simulink model "uz_3ph_ParameterID"  (R2022b)
settings: Solver=FixedStepDiscrete  StartTime=0.0  StopTime=160  FixedStep=0.000005  RelTol=1e-3  EnableMultiTasking=on
model workspace (MATLAB code in the model file):
  | cmdLim = Simulink.Parameter;
  | cmdLim.Value = 15;
  | cmdLim.Description = 'Limit for controlling the maximum surface command angle.';
  | cmdLim.Min = 0;
  | cmdLim.Max = 90;
  | cmdLim.DocUnits = 'deg';
  | 
  | dispGain = Simulink.Parameter;
  | dispGain.Value = 0.75;
  | dispGain.Description = 'Gain applied to the displacement error.';
  | dispGain.Min = 0;
  | dispGain.Max = [];
  | dispGain.DocUnits = 'deg/sec/deg';
  | 
  | dispLim = Simulink.Parameter;
  | dispLim.Value = 30;
  | dispLim.Description = 'Limit for controlling the maximum commanded angle.';
  | dispLim.Min = 0;
  | dispLim.Max = 180;
  | dispLim.DocUnits = 'deg';
  | 
  | intGain = Simulink.Parameter;
  | intGain.Value = 0.5;
  | intGain.Description = 'Gain applied to the integral error.';
  | intGain.Min = 0;
  | intGain.Max = [];
  | intGain.DocUnits = 'deg/sec/deg/sec';
  | 
  | intLim = Simulink.Parameter;
  | intLim.Value = 5;
  | intLim.Description = 'Limit for controlling the maximum commanded angle.';
  | intLim.Min = 0;
  | intLim.Max = 90;
  | intLim.DocUnits = 'deg';
  | 
  | rateGain = Simulink.Parameter;
  | rateGain.Value = 2;
  | rateGain.Description = 'Gain applied to the rate error.';
  | rateGain.Min = 0;
  | rateGain.Max = [];
  | rateGain.DocUnits = 'deg/deg/sec';
  | 
  | rateLim = Simulink.Parameter;
  | rateLim.Value = 6;
  | rateLim.Description = 'Limit for controlling the maximum commanded angle.';
  | rateLim.Min = 0;
  | rateLim.Max = 180;
  | rateLim.DocUnits = 'deg/sec';
  | 
  | hdgGain = Simulink.Parameter;
  | hdgGain.Value = 0.015;
values from neighbouring files (symbols this model uses):
  d_d_TMS = 0.005    [Parameter_Init_Buehler_201.m]
  d_f_hardware = 200000    [Parameter_Init_Buehler_201.m]
  d_f_states = 20000    [Parameter_Init_Buehler_201.m]
  d_i_max = 15    [Parameter_Init_Buehler_201.m]
  d_i_min = -d_i_max    (= -15)    [Parameter_Init_Buehler_201.m]
  d_I_n = 8    [Parameter_Init_Buehler_201.m]
  d_J_Coupling_M_E = 2e-6    (= 2e-06)    [Parameter_Init_Buehler_201.m]
  d_J_Coupling_M_Ms = 2e-20    [Parameter_Init_Buehler_201.m]
  d_J_Ms_L = d_J_Ms_M    (= 1.26363648e-05)    [Parameter_Init_Buehler_201.m]
  d_J_Ms_M = 0.5*0.5*((0.5*d_d_Ms)^4)*3.14*d_l_Ms*d_rho_Ms    (= 1.26363648e-05)    [Parameter_Init_Buehler_201.m]
  d_L_d = 0.00031    [Parameter_Init_Buehler_201.m]
  d_L_q = 0.00033    [Parameter_Init_Buehler_201.m]
  d_p = 4    [Parameter_Init_Buehler_201.m]
  d_psi_pm = 0.0075    [Parameter_Init_Buehler_201.m]
  d_R_ph = d_R_ph_ph/2    (= 0.089)    [Parameter_Init_Buehler_201.m]
  d_y_max = 10    [Parameter_Init_Buehler_201.m]
  d_y_min = -d_y_max    (= -10)    [Parameter_Init_Buehler_201.m]
undefined symbols (not defined in the file or in its folder): i_dq, i_dq_ref, n_ref, V_abc, v_dq
libraries: fl_lib x47, nesl_utility x30, ee_lib x18, simulink x8, spsabctodq0Lib x2, spsdq0toabcLib x1, spsTriangleGeneratorLib x1
(part 1 of 4)
settings Model: RequirementInfo={} %GIDa_fe9045fd_0412_4b6e_8206_617cc20e6fde  FPTRunName=Active  Creator=ts  LastModifiedBy=valen
settings SolverCC: AlgebraicLoopSolver=TrustRegion  PositivePriorityOrder=on  AutoInsertRateTranBlk=on
settings DataIOCC: SaveOutput=off  SignalLogging=off  DSMLogging=off  SaveTime=off
settings OptimizationCC: DefaultParameterBehavior=Inlined  UseDivisionForNetSlopeComputation=on  GainParamInheritBuiltInType=on  UseFloatMulNetSlope=on  DefaultUnderspecifiedDataType=single  UseSpecifiedMinMax=on  InlineInvariantSignals=on  PassReuseOutputArgsAs=Individual arguments  ZeroExternalMemoryAtStartup=off  ZeroInternalMemoryAtStartup=off  NoFixptDivByZeroProtection=on  EfficientFloat2IntCast=on  LifeSpan=1  MaxStackSize=64  OptimizeBlockOrder=speed  DifferentSizesBufferReuse=on  EfficientTunableParamExpr=on
settings DebuggingCC: UnconnectedInputMsg=warning  UnconnectedOutputMsg=warning  UnconnectedLineMsg=warning  BusObjectLabelMismatch=error  AllowSymbolicDim=off  SFUnexpectedBacktrackingDiag=warning  SFNoUnconditionalDefaultTransitionDiag=warning  SFExecutionAtInitializationDiag=none  SFMachineParentedDataDiag=warning  ArithmeticOperatorsInVariantConditions=warning
settings HardwareCC: ProdBitPerPointer=32  ProdBitPerSizeT=32  ProdBitPerPtrDiffT=32  ProdLargestAtomicInteger=Long  ProdLargestAtomicFloat=Double  ProdWordSize=32  ProdLongLongMode=on  ProdHWDeviceType=ARM Compatible->ARM Cortex-R  HardwareBoardFeatureSet=SoCBlockset
settings ModelReferenceCC: EnableRefExpFcnMdlSchedulingChecks=on
settings SFSimCC: SimGenImportedTypeDefs=on  MATLABDynamicMemAlloc=off
settings RTWCC: Description=Embedded Coder  SystemTargetFile=ert.tlc  GenCodeOnly=on  TemplateMakefile=ert_default_tmf  GenerateReport=on  BuildConfiguration=Faster Runs  IncludeHyperlinkInReport=on  LaunchReport=on  GenerateTraceInfo=on  GenerateTraceReport=on  GenerateTraceReportSl=on  GenerateTraceReportSf=on  GenerateTraceReportEml=on  GenerateCodeMetricsReport=on  CheckMdlBeforeBuild=Warning  DLArmComputeVersion=19.05
settings CodeAppCC: ForceParamTrailComments=on  IgnoreCustomStorageClasses=off  OperatorAnnotations=on  SimulinkDataObjDesc=on  SFDataObjDesc=on  MATLABFcnDesc=on  CustomSymbolStrGlobalVar=rt$M$R$N  CustomSymbolStrType=$N$M$R_t  CustomSymbolStrFcn=$N$M$F  CustomSymbolStrMacro=$N$M  InsertBlockDesc=on  StateflowObjectComments=on  MATLABSourceComments=on  EnableCustomComments=on  ReqsInCode=on
settings ERTTargetCC: TargetLangStandard=C99 (ISO)  CodeReplacementLibrary=GNU C99 extensions  MultiwordLength=2048  IncludeMdlTerminateFcn=off  CombineSignalStateStructs=on  SuppressErrorStatus=on  IncludeFileDelimiter=UseQuote  CodeInterfacePackaging=Reusable function  SupportNonFinite=off  RemoveResetFunc=off  InlinedParameterPlacement=NonHierarchical  MultiInstanceErrorCode=Warning  RootIOFormat=Part of model data structure  ERTCustomFileTemplate=example_file_process.tlc  GlobalDataDefinition=InSourceFile  GlobalDataReference=InSourceFile  ERTFilePackagingFormat=CompactWithDataFile  SuppressUnreachableDefaultCases=off
settings ConfigComp: CovScope=ReferencedModels  CovSaveName=covdata_rollAP  CovMetricSettings=dcmtrwe  CovHTMLOptions=-sRT=1 -aTS=1 -bRG=1 -bTC=1 -hTR=1 -nFC=0 -scm=1 -bcm=1 -xEv=0  CovSaveCumulativeToWorkspaceVar=on  CovSaveSingleToWorkspaceVar=on  CovCumulativeVarName=covCumulativeData_rollAP  CovReportOnPause=off  CovExternalEMLEnable=off  CovSFcnEnable=off

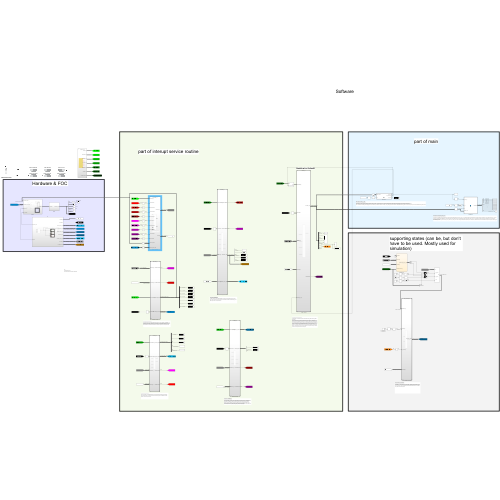
[thumbnail: Simulink's stored preview of the top-level diagram]
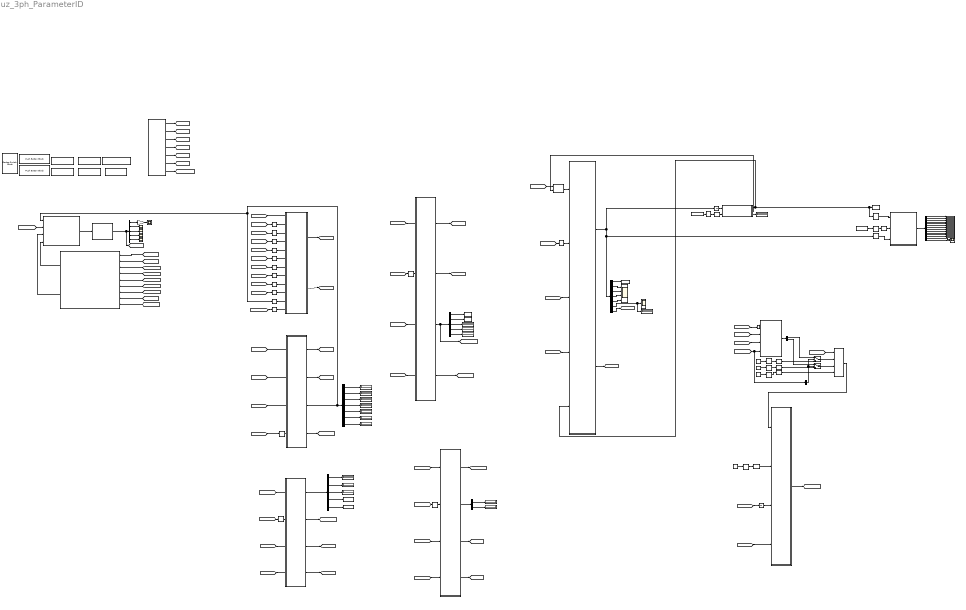
== system uz_3ph_ParameterID ==
  note: todo:
      | -control state reference
      | -two mass generieren mit externen definitionen
  note: Description of Interpoaltion_Mesh_Grid:
      |
      | This function is calculating the regular flux maps out of the irregular scatter data array stored in psi_array_in. The outputs rangeX are containg the flux maps axis information, whereby the range is related to 3 times "i_rat" input.
      | Furthermore, the temperature dependency of the permanent flux is calculated if there are enough measuring values stored in the "delta_psi" array. The temperature constant as well as the estimated error of permanent flux,
      | at reference temperature, are given out on "psi_temp_const" and "psi_temp_error" outputs. Using this temperature dependency, the flux maps are updated with the permanent flux offset caused by the temperature which is given
      | in on "Wtemp_in" input.
  note: Stateflow for OnlineID
  note: part of main
  note: part of interupt service routine
  note: Software
  note: Hardware & FOC
  note: Description of clean_psi_array:
      |
      | This function is cleaning the array storing the measurement values, which always consits of a d-q-current combination a winding temperature and a speed value such as a d-q-flux combination
      | The function is searching for measuring pairs which are closer than "eta_c" to their neighbours. In this case it is averaging this similar pairs to avoid measuring values containing the same information.
      | This is essential for calculating a wide ranging flux map out of this array. Furthermore, there is an output "n_flux_points" giving back the amount of independent measuring pairs. This is the number (x/100) i show in the JavaGUI on the rigth top corner.
  note: Description of ElectricalID:
      |
      | This state includes an automated identification process for typical parameters of a PMSM. This includes the identification of the polepairs, theta_offset of a incremental encoder, Rs, Ld, Lq, Psi_PM and J. The control parameters of a FOC will be calculated with the identified parameters and are therefore tuned for the used machine. This state requires some sort of speed control.
  note: Description OnlineID Stateflow:
      |
      | This Stateflow is used to detect special transient states and to gather measuring data in these states.
      | This is done to identify the parameters of the linear pmsm model. This includes Rs, Ld, Lq and Psi_PM. The flux maps can be identified aswell. With each new operating point the relevant signals are measured and the flux in the specific operating point is calculated. Up to 100 unique values will be stored in an array, which will later be cleaned up with external functions. In contrast to the FluxMapID state, this state does not actively control the machine via reference currents(except the addition of a injection signal with low amplitude/frequency on top of the reference d-axis current), but therefore measures and calculates the flux in the operating points. This state can therefore run in parallel with your controller, since it does not require full control of the system.
  note: Description of FrictionID:
      |
      | This state includes an automated identification process for different friction/torque parameters. The breakaway torque, coloumb torque and viscous friction torque will be identified. This state requires some sort of speed control.
  note: Description of FluxMapID:
      |
      | This state includes an process for FluxMap identification. The desired range of the identified flux maps can be set in the d- and q-axis, with an input for the stepsize aswell. From these input parameters, this state will create a rectangular grid. Each point of this grid will be set and reference currents outputed to an external current controller. This state needs some sort of current controller to work properly. It does NOT measure the needed signals to calculate the flux maps in each point. It only controls the triggering of the operating points.
  note: Description of TwoMassID:
      |
      | This state includes an automated identification process for typical parameters of a two mass system. This includes the inertia of the motor and load side, the stiffness and the damping. This state requires some sort of speed control.
  note: Description FOC_ControlState:
      |
      | This Stateflow is entered, after every other ID-state is finished (except OnlineID). It's just a simple state for current & speed control, depending on what the user chose in the config. This is only used to control the FOC with inputs after the ID-states are done. This state is solely used for simulation purposes.
  note: supporting states (can be, but don't have to be used. Mostly used for simulation)
  0 = current control 1 = speed control : Constant
  AutoRefCurrents : Stateflow chart  TreatAsAtomicUnit=on
      settings: PortSchema="{\"entries\":[{\"content\":{\"sides\":[{\"content\":{\"connectorIds\":[\"In1\",\"In2\",\"In4\",\"In3\"]},\"type\":\"ConnectorPlacement.EquallySpacedRectSide\",\"uuid\":\"72ec0a24-315d-4dd0-9768-288ce3b452e0\"},{\"content\":{\"connectorIds\":[\"Out1\"],\"side\":\"RIGHT\"},\"type\":\"ConnectorPlacement.EquallySpacedRectSide\",\"uuid\":\"ab2b6233-d9cb-4afd-91e6-1fd664e04fd4\"},{\"content\":{\"connectorIds\":[],\"side\":\"TOP\"},\"type\":\"ConnectorPlacement.EquallySpacedRectSide\",\"uuid\":\"64b2df27-0928-499d-b44c-d4351b3511f9\"}]},\"type\":\"ConnectorPlacement.EquallySpacedConnector\",\"uuid\":\"4bb55e1f-14f7-4ef2-bb52-ee940a9b3e5d\"}],\"packageUris\":[\"http://schema.mathworks.com/mf0/Connector/R2020b\"],\"version\":\"1.0\"}"
  Bus Assignment : BusAssignment  AssignedSignals=i_dq_ref.d,i_dq_ref.q,n_ref
  Bus Assignment1 : BusAssignment  AssignedSignals=array_cleaned
  Bus Selector : BusSelector  OutputSignals=BrkTorque,CoulTorque,ViscoTorque,measArrayTorque,measArraySpeed
  Bus Selector1 : BusSelector  OutputSignals=omega_m,i_dq,v_dq,I_abc,V_abc
  Bus Selector2 : BusSelector  OutputSignals=thetaOffset,PMSM_parameters.R_ph_Ohm,PMSM_parameters.Ld_Henry,PMSM_parameters.Lq_Henry,PMSM_parameters.Psi_PM_Vs,PMSM_parameters.J_kg_m_squared,PMSM_parameters.polePairs
  Bus Selector3 : BusSelector  OutputSignals=range_psid_X,range_psiq_X,range_id_X,range_iq_X,range_psid_Y,range_psiq_Y,range_id_Y,range_iq_Y,psiq_grid,psid_grid,id_grid,iq_grid,psi_temp_const,psi_temp_error
  Bus Selector4 : BusSelector  OutputSignals=i_dq_ref.d,i_dq_ref.q
  Bus Selector5 : BusSelector  OutputSignals=R_s,WindingTemp
  Bus Selector6 : BusSelector  OutputSignals=c_est_out,d_est_out,LoadInertia,TrainInertia,rotorInertia
  Bus Selector7 : BusSelector  OutputSignals=enableCRS
  Bus Selector8 : BusSelector  OutputSignals=psi_array,Rph_out,Ld_out,Lq_out,psi_pm_out,activeState,id_out
  CleanPsiArray : MATLAB Function
  Const27 : Constant  Value=0.01*d_I_n
  Const53 : Constant  Value=d_I_n
  Const7 : Constant  Value=0.6
  Const8 : Constant  Value=0
  Const9 : Constant  Value=1000
  Data Type Conversion107 : DataTypeConversion  OutDataTypeStr=boolean  SaturateOnIntegerOverflow=off  RndMeth=Floor
  Data Type Conversion{12..13,15,60,86} (5 alike) : DataTypeConversion  OutDataTypeStr=single  SaturateOnIntegerOverflow=off  RndMeth=Floor
  Delay{,1..9,14} (11 alike) : Delay  DelayLength=1  InitialCondition=0
  Display{1..3,5..11} (10 alike) : Display
  ElectricalID_subsystem : ModelReference  ModelNameDialog=ElectricalID_ref.slx  SimulationMode=Normal  ModelReferenceVersion=5.61
      settings: PortSchema="{\"entries\":[{\"content\":{\"sides\":[{\"content\":{\"connectorIds\":[\"In3\",\"In4\",\"In1\",\"In2\"]},\"type\":\"ConnectorPlacement.EquallySpacedRectSide\",\"uuid\":\"f0ac0bcf-14d9-46a0-98b5-cf926ef17a03\"},{\"content\":{\"connectorIds\":[\"Out1\",\"Out2\",\"Out4\",\"Out3\"],\"side\":\"RIGHT\"},\"type\":\"ConnectorPlacement.EquallySpacedRectSide\",\"uuid\":\"3432f655-d87e-4f4a-bc13-594c8277a670\"},{\"content\":{\"connectorIds\":[],\"side\":\"TOP\"},\"type\":\"ConnectorPlacement.EquallySpacedRectSide\",\"uuid\":\"598e67a2-ee08-4059-aaa7-0b5cb688c228\"}]},\"type\":\"ConnectorPlacement.EquallySpacedConnector\",\"uuid\":\"e19c3dd0-4872-4ea8-9ebd-fc7e1d9ddc42\"}],\"packageUris\":[\"http://schema.mathworks.com/mf0/Connector/R2020b\"],\"version\":\"1.0\"}"
  FOC : Subsystem
  FOC_ControlState_subsystem : ModelReference  ModelNameDialog=FOC_ControlState_ref.slx  SimulationMode=Normal  ModelReferenceVersion=5.47
      settings: PortSchema="{\"entries\":[{\"content\":{\"sides\":[{\"content\":{\"connectorIds\":[\"In2\",\"In4\",\"In1\",\"In3\"]},\"type\":\"ConnectorPlacement.EquallySpacedRectSide\",\"uuid\":\"51616e24-a97c-4867-a832-fbf8995ba5af\"},{\"content\":{\"connectorIds\":[\"Out1\"],\"side\":\"RIGHT\"},\"type\":\"ConnectorPlacement.EquallySpacedRectSide\",\"uuid\":\"f89ef2d6-1fe7-4143-9573-492fc01180c7\"},{\"content\":{\"connectorIds\":[],\"side\":\"TOP\"},\"type\":\"ConnectorPlacement.EquallySpacedRectSide\",\"uuid\":\"2a1663ee-9e4b-4188-8f87-b811d0bf4173\"}]},\"type\":\"ConnectorPlacement.EquallySpacedConnector\",\"uuid\":\"7415555a-a8a9-4dd7-91ae-86382220971a\"}],\"packageUris\":[\"http://schema.mathworks.com/mf0/Connector/R2020b\"],\"version\":\"1.0\"}"
  FluxMapID_subsystem : ModelReference  ModelNameDialog=FluxMapID_ref.slx  SimulationMode=Normal  ModelReferenceVersion=5.45
      settings: PortSchema="{\"entries\":[{\"content\":{\"sides\":[{\"content\":{\"connectorIds\":[\"In1\",\"In2\",\"In3\",\"In4\"]},\"type\":\"ConnectorPlacement.EquallySpacedRectSide\",\"uuid\":\"981d5bbf-03cd-4404-8840-685ce2b7a497\"},{\"content\":{\"connectorIds\":[\"Out3\",\"Out4\",\"Out1\",\"Out2\"],\"side\":\"RIGHT\"},\"type\":\"ConnectorPlacement.EquallySpacedRectSide\",\"uuid\":\"92ae37cc-cac4-4d7b-af20-0fade983881b\"},{\"content\":{\"connectorIds\":[],\"side\":\"TOP\"},\"type\":\"ConnectorPlacement.EquallySpacedRectSide\",\"uuid\":\"d233b8d0-893b-4073-8e4e-3204ab89fedb\"}]},\"type\":\"ConnectorPlacement.EquallySpacedConnector\",\"uuid\":\"28ed47dd-3acf-49aa-8a06-7eb7a90c4cf1\"}],\"packageUris\":[\"http://schema.mathworks.com/mf0/Connector/R2020b\"],\"version\":\"1.0\"}"
  FrictionID_subsystem : ModelReference  ModelNameDialog=FrictionID_ref.slx  SimulationMode=Normal  ModelReferenceVersion=5.45
      settings: PortSchema="{\"entries\":[{\"content\":{\"sides\":[{\"content\":{\"connectorIds\":[\"In1\",\"In2\",\"In3\",\"In4\"]},\"type\":\"ConnectorPlacement.EquallySpacedRectSide\",\"uuid\":\"9228c284-4dde-45fc-9186-6f631f78e5bf\"},{\"content\":{\"connectorIds\":[\"Out4\",\"Out3\",\"Out2\",\"Out1\"],\"side\":\"RIGHT\"},\"type\":\"ConnectorPlacement.EquallySpacedRectSide\",\"uuid\":\"71961043-480b-43aa-8cdd-23d9057d5ad4\"},{\"content\":{\"connectorIds\":[],\"side\":\"TOP\"},\"type\":\"ConnectorPlacement.EquallySpacedRectSide\",\"uuid\":\"f6f3bc9d-566f-4498-bf43-24e8b901b7a7\"}]},\"type\":\"ConnectorPlacement.EquallySpacedConnector\",\"uuid\":\"83d2d7c4-30d1-4ed4-b102-cbae6a0e9817\"}],\"packageUris\":[\"http://schema.mathworks.com/mf0/Connector/R2020b\"],\"version\":\"1.0\"}"
  Gain : Gain  Gain=60/(2*pi)
  Hardware : Subsystem
  I_abc : Scope
  InterpMeshGrid : MATLAB Function  TreatAsAtomicUnit=on
  OnlineActiveState : Scope
  OnlineID_subsystem : ModelReference  ModelNameDialog=OnlineID_ref.slx  SimulationMode=Normal  ModelReferenceVersion=5.46
      settings: PortSchema="{\"entries\":[{\"content\":{\"sides\":[{\"content\":{\"connectorIds\":[\"In2\",\"In3\",\"In4\",\"In5\",\"In1\"]},\"type\":\"ConnectorPlacement.EquallySpacedRectSide\",\"uuid\":\"7820c6f2-c977-4194-b662-7782d124a170\"},{\"content\":{\"connectorIds\":[\"Out1\",\"Out2\"],\"side\":\"RIGHT\"},\"type\":\"ConnectorPlacement.EquallySpacedRectSide\",\"uuid\":\"8a942b25-9a71-4f6d-9e71-d8e23af023a4\"},{\"content\":{\"connectorIds\":[],\"side\":\"TOP\"},\"type\":\"ConnectorPlacement.EquallySpacedRectSide\",\"uuid\":\"547238ca-03bf-4702-a4be-178f97463404\"}]},\"type\":\"ConnectorPlacement.EquallySpacedConnector\",\"uuid\":\"69f1930a-cf81-42da-9647-066ad6599903\"}],\"packageUris\":[\"http://schema.mathworks.com/mf0/Connector/R2020b\"],\"version\":\"1.0\"}"
  Push Button2 : PushButtonBlock  ButtonText=RESET
  Push Button3 : PushButtonBlock  ButtonText=ACCEPT  OffValue=1.000000
  RT : RateTransition  OutPortSampleTime=0.0001
  Rate Transition : RateTransition  OutPortSampleTime=0.1
  Rate Transition{1..6,13..14,78,147} (10 alike) : RateTransition  OutPortSampleTime=1/d_f_states
  Rate Transition85 : RateTransition  OutPortSampleTime=0.1
  Rate Transition90 : RateTransition  OutPortSampleTime=0.1
  Rs,Ld,Lq,Psi_pm : Scope  NumInputPorts=4
  Scope2 : Scope  NumInputPorts=2
  Select Control : SliderSwitchBlock  LabelPosition=Hide
      settings: Values={{'Current', 'Speed'}, [0 1]}
  Subsystem Reference : Subsystem  ReferencedSubsystem=model_bus_init
  Subsystem Reference1 : Subsystem  ReferencedSubsystem=ControlState_ref
  Switch2 : Switch  Criteria=u2 > Threshold  SaturateOnIntegerOverflow=off  InputSameDT=off
  Switch3 : Switch  Criteria=u2 > Threshold  SaturateOnIntegerOverflow=off  InputSameDT=off
  To Workspace1 : ToWorkspace  VariableName=measArrayTorque  SampleTime=-1
      settings: MaxDataPoints=1
  To Workspace15 : ToWorkspace  VariableName=psi_array_cleaned  SampleTime=-1
      settings: MaxDataPoints=1
  To Workspace16 : ToWorkspace  VariableName=rangepdX  SampleTime=-1
      settings: MaxDataPoints=1
  To Workspace17 : ToWorkspace  VariableName=rangepqX  SampleTime=-1
      settings: MaxDataPoints=1
  To Workspace18 : ToWorkspace  VariableName=rangeidX  SampleTime=-1
      settings: MaxDataPoints=1
  To Workspace19 : ToWorkspace  VariableName=rangeiqX  SampleTime=-1
      settings: MaxDataPoints=1
  To Workspace2 : ToWorkspace  VariableName=measArraySpeed  SampleTime=-1
      settings: MaxDataPoints=1
  To Workspace20 : ToWorkspace  VariableName=rangepdY  SampleTime=-1
      settings: MaxDataPoints=1
  To Workspace21 : ToWorkspace  VariableName=rangepqY  SampleTime=-1
      settings: MaxDataPoints=1
  To Workspace22 : ToWorkspace  VariableName=rangeidY  SampleTime=-1
      settings: MaxDataPoints=1
  To Workspace23 : ToWorkspace  VariableName=rangeiqY  SampleTime=-1
      settings: MaxDataPoints=1
  To Workspace24 : ToWorkspace  VariableName=psiq_grid  SampleTime=-1
      settings: MaxDataPoints=1
  To Workspace25 : ToWorkspace  VariableName=psid_grid  SampleTime=-1
      settings: MaxDataPoints=1
  To Workspace26 : ToWorkspace  VariableName=id_grid  SampleTime=-1
      settings: MaxDataPoints=1
  To Workspace27 : ToWorkspace  VariableName=iq_grid  SampleTime=-1
      settings: MaxDataPoints=1
  To Workspace3 : ToWorkspace  VariableName=psi_array  SampleTime=-1
      settings: MaxDataPoints=1
  To Workspace31 : ToWorkspace  VariableName=c_est_out  SampleTime=-1
      settings: MaxDataPoints=1
  To Workspace32 : ToWorkspace  VariableName=d_est_out  SampleTime=-1
      settings: MaxDataPoints=1
  TwoMassID_subsystem : ModelReference  ModelNameDialog=TwoMassID_ref.slx  SimulationMode=Normal  ModelReferenceVersion=5.45
      settings: PortSchema="{\"entries\":[{\"content\":{\"sides\":[{\"content\":{\"connectorIds\":[\"In1\",\"In2\",\"In3\",\"In4\"]},\"type\":\"ConnectorPlacement.EquallySpacedRectSide\",\"uuid\":\"b3f846b4-67b8-414d-80f8-2cdf230e8050\"},{\"content\":{\"connectorIds\":[\"Out1\",\"Out2\",\"Out4\",\"Out3\"],\"side\":\"RIGHT\"},\"type\":\"ConnectorPlacement.EquallySpacedRectSide\",\"uuid\":\"f153ecc1-7a63-46b5-bb71-72b88e4117b7\"},{\"content\":{\"connectorIds\":[],\"side\":\"TOP\"},\"type\":\"ConnectorPlacement.EquallySpacedRectSide\",\"uuid\":\"7aaf7a4c-17fe-4dd1-8ce1-675b09504e17\"}]},\"type\":\"ConnectorPlacement.EquallySpacedConnector\",\"uuid\":\"e21480e7-4483-4a1e-b62d-5327482c3f88\"}],\"packageUris\":[\"http://schema.mathworks.com/mf0/Connector/R2020b\"],\"version\":\"1.0\"}"
  Unit Delay : UnitDelay  SampleTime=-1  HasFrameUpgradeWarning=on
  Unit Delay3 : UnitDelay  SampleTime=-1  HasFrameUpgradeWarning=on
  V_abc : Scope
  d-axis inductance Ld [H] : Display
  dqTrans : Subsystem
  enable ElectricalID : SliderSwitchBlock  LabelPosition=Hide
      settings: Values={{'Off', 'On'}, [0 1]}
  enable FluxMapID : SliderSwitchBlock  LabelPosition=Hide
      settings: Values={{'Off', 'On'}, [0 1]}
  enable FrictionID : SliderSwitchBlock  LabelPosition=Hide
      settings: Values={{'Off', 'On'}, [0 1]}
  enable OnlineID : SliderSwitchBlock  LabelPosition=Hide
      settings: Values={{'Off', 'On'}, [0 1]}
  enable TwoMassID : SliderSwitchBlock  LabelPosition=Hide
      settings: Values={{'Off', 'On'}, [0 1]}
  enableParameterID : RockerSwitchBlock  LabelPosition=Hide
      settings: Values={{'Off', 'On'}, [0 1]}
  i_d i_q : Scope
  p : Display
  phase resistance [Ohm] : Display
  psiPM [Vs] : Display
  q-axis inductance Lq [H] : Display
  rotor speed [rpm] : Scope
  rotorInertia  [kg*m²] : Display
  thetaOffset [rad] : Display
  v_d v_q : Scope
  wires:
  FrictionID_subsystem/1 -> [finishedFrictionID]
  Bus Selector/3 -> Display10/1  "<ViscoTorque>"
  FluxMapID_subsystem/1 -> [finishedFluxMapID]
  [ControlFlags] -> OnlineID_subsystem/5
  Const8/1 -> Rate Transition13/1
  Subsystem Reference/5 -> [TwoMassIDConfig]
  Bus Selector2/4 -> q-axis inductance Lq [H]/1  "<Lq_Henry>"
  [GlobalConfig] -> AutoRefCurrents/2(GlobalConfig)
  [GlobalConfig] -> FluxMapID_subsystem/3
  [finishedFrictionID] -> Delay/1
  Rate Transition5/1 -> FrictionID_subsystem/2
  TwoMassID_subsystem/4 -> [TwoMassID_output], Bus Selector6/1
  OnlineID_subsystem/1 -> Bus Selector8/1, Rate Transition90/1, Unit Delay3/1
  Bus Selector2/5 -> psiPM [Vs]/1  "<Psi_PM_Vs>"
  Gain/1 -> rotor speed [rpm]/1
  Bus Selector8/2 -> Rs,Ld,Lq,Psi_pm/1  "<Rph_out>"
  Rate Transition2/1 -> TwoMassID_subsystem/2
  ElectricalID_subsystem/3 -> [ElectricalID_FOC_output]
  Bus Selector6/5 -> Display6/1  "<rotorInertia>"
  Const9/1 -> Rate Transition1/1
  Rate Transition14/1 -> Data Type Conversion13/1
  Subsystem Reference/1 -> [GlobalConfig_in]
  ElectricalID_subsystem/4 -> Hardware/1(ElectricalID_output), Delay14/1, Bus Selector2/1
  [FrictionIDConfig] -> FrictionID_subsystem/1
  [FluxMapID_FOC_output] -> FOC/5(FluxMapID_FOC_input)
  [enteredElectricalID] -> Delay5/1
  ElectricalID_subsystem/1 -> [enteredElectricalID]
  Rate Transition85/1 -> Data Type Conversion86/1
  [enteredFrictionID] -> Delay1/1
  [FOCControl_output] -> FOC/6(FOCControl_input)
  FluxMapID_subsystem/4 -> Bus Selector5/1
  Data Type Conversion13/1 -> Switch2/3  "i_q_ref"
  Rate Transition90/1 -> InterpMeshGrid/3(OnlineID_input)
  [finishedFluxMapID] -> Delay4/1
  ElectricalID_subsystem/2 -> [finishedElectricalID]
  [ControlFlags] -> ElectricalID_subsystem/4
  [finishedTwoMassID] -> Delay3/1
  FOC/2(PWM_out) -> Hardware/3(PWM_FOC_in)
  [ActualValues] -> RT/1
  Bus Selector1/1 -> Gain/1  "<omega_m>"
  Subsystem Reference/2 -> [ElectricalIDConfig]
  [ElectricalIDConfig] -> ElectricalID_subsystem/1
  TwoMassID_subsystem/3 -> [TwoMassID_FOC_output]
  Subsystem Reference/4 -> [FrictionIDConfig]
  Const53/1 -> Rate Transition85/1
  [GlobalConfig] -> TwoMassID_subsystem/3
  FluxMapID_subsystem/3 -> [FluxMapID_FOC_output]
  Const27/1 -> Rate Transition78/1
  [ControlFlags] -> TwoMassID_subsystem/4
  TwoMassID_subsystem/1 -> [finishedTwoMassID]
  Data Type Conversion60/1 -> CleanPsiArray/2(eta_c)
  Bus Selector2/6 -> rotorInertia  [kg*m²]/1  "<J_kg_m_squared>"
  Bus Selector/1 -> Display11/1  "<BrkTorque>"
  [TwoMassIDConfig] -> TwoMassID_subsystem/1
  Bus Selector2/7 -> p/1  "<polePairs>"
  [ElectricalID_FOC_output] -> Delay8/1
  Rate Transition13/1 -> Data Type Conversion12/1
  Unit Delay/1 -> FOC_ControlState_subsystem/1
  FrictionID_subsystem/3 -> [FrictionID_FOC_output]  "FrictionID_FOC_output"
  Rate Transition/1 -> InterpMeshGrid/1(psi_array_in)
  TwoMassID_subsystem/2 -> [enteredTwoMassID]
  Bus Selector2/2 -> phase resistance [Ohm]/1  "<R_ph_Ohm>"
  Rate Transition3/1 -> OnlineID_subsystem/3
  [GlobalConfig] -> ElectricalID_subsystem/3
  Bus Selector2/3 -> d-axis inductance Ld [H]/1  "<Ld_Henry>"
  [ActualValues] -> Rate Transition6/1
  Bus Selector6/3 -> Display3/1  "<LoadInertia>"
  [ControlFlags] -> FOC/1(ControlFlags)
  Rate Transition6/1 -> ElectricalID_subsystem/2
  [FluxMapIDConfig] -> FluxMapID_subsystem/1
  [ActualValues] -> Rate Transition2/1
  Subsystem Reference/6 -> [OnlineIDConfig]
  [ControlFlags] -> FluxMapID_subsystem/4
  [ActualValues] -> Rate Transition3/1
  CleanPsiArray/2(array_cleaned_flag) -> Bus Assignment1/2
  Bus Selector5/1 -> Display1/1  "<R_s>"
  [GlobalConfig] -> FrictionID_subsystem/3
  [ControlFlags] -> FOC_ControlState_subsystem/3
  [ElectricalID_FOC_output] -> Hardware/2(ElectricalID_FOC_output)
  Const7/1 -> Rate Transition14/1
  FrictionID_subsystem/4 -> Bus Selector/1
  FrictionID_subsystem/2 -> [enteredFrictionID]
  Bus Selector6/4 -> Display5/1  "<TrainInertia>"
  Hardware/1(ActualValues) -> dqTrans/1(ActualValues)
  Data Type Conversion86/1 -> InterpMeshGrid/2(i_rat)
  Bus Selector8/5 -> Rs,Ld,Lq,Psi_pm/4  "<psi_pm_out>"
  Bus Selector8/3 -> Rs,Ld,Lq,Psi_pm/2  "<Ld_out>"
  Unit Delay3/1 -> CleanPsiArray/1(OnlineID_output)
  [OnlineIDConfig] -> Bus Assignment1/1
  [TwoMassID_FOC_output] -> FOC/7(TwoMassID_FOC_input)
  Rate Transition78/1 -> Data Type Conversion60/1
  Rate Transition1/1 -> Data Type Conversion15/1
  Bus Selector8/6 -> Display8/1, OnlineActiveState/1  "<activeState>"
  CleanPsiArray/1(psi_array_out) -> Rate Transition/1, To Workspace15/1, OnlineID_subsystem/1  "cleaned_psi_array"
  [GlobalConfig] -> OnlineID_subsystem/4
  FOC/1(FOC_enable_out) -> Hardware/4(FOC_enabled)
  Bus Selector2/1 -> thetaOffset [rad]/1  "<thetaOffset>"
  Rate Transition4/1 -> FluxMapID_subsystem/2
  Subsystem Reference/3 -> [FluxMapIDConfig]
  [FrictionID_FOC_output] -> FOC/3(FrictionID_FOC_input)
  Bus Selector1/2 -> i_d i_q/1  "<i_dq>"
  CleanPsiArray/3(n_flux_points) -> Display7/1
  Bus Selector/2 -> Display9/1  "<CoulTorque>"
  FluxMapID_subsystem/2 -> [enteredFluxMapID]
  [ActualValues] -> Rate Transition4/1
  Bus Selector6/1 -> To Workspace31/1  "<c_est_out>"
  Bus Selector6/2 -> To Workspace32/1  "<d_est_out>"
  FOC_ControlState_subsystem/1 -> [FOCControl_output]
  [finishedElectricalID] -> Delay7/1
  [ElectricalID_FOC_output] -> FOC/4(ElectricalID_FOC_input)
  Bus Assignment/1 -> FOC_ControlState_subsystem/2
  [ControlFlags] -> FrictionID_subsystem/4
  [ActualValues] -> Rate Transition5/1
  Bus Selector8/4 -> Rs,Ld,Lq,Psi_pm/3  "<Lq_out>"
  Data Type Conversion12/1 -> Switch3/3  "i_d_ref"
  [enteredFluxMapID] -> Delay2/1
  [ActualValues] -> FOC/2(ActualValues)
  [enteredTwoMassID] -> Delay6/1
  Bus Selector5/2 -> Display2/1  "<WindingTemp>"
  Bus Selector1/3 -> v_d v_q/1  "<v_dq>"
  Bus Selector1/4 -> I_abc/1  "<I_abc>"
  Bus Selector1/5 -> V_abc/1  "<V_abc>"
  [GlobalConfig] -> Bus Assignment/1
  Switch2/1 -> Bus Assignment/3
  Switch3/1 -> Bus Assignment/2
  Data Type Conversion15/1 -> Bus Assignment/4  "n_ref"
  RT/1 -> AutoRefCurrents/1(ActualValues)
  Bus Selector8/7 -> [OnlineID_id_out]  "<id_out>"
  [OnlineID_id_out] -> Unit Delay/1
  Rate Transition147/1 -> Data Type Conversion107/1
  Data Type Conversion107/1 -> FOC_ControlState_subsystem/4  "controlType"
  0 = current control 1 = speed control/1 -> Rate Transition147/1
  Bus Assignment1/1 -> OnlineID_subsystem/2
  Bus Selector3/1 -> To Workspace16/1  "<range_psid_X>"
  Bus Selector3/2 -> To Workspace17/1  "<range_psiq_X>"
  InterpMeshGrid/1(FluxMapData) -> Bus Selector3/1
  Bus Selector3/14 -> Scope2/2  "<psi_temp_error>"
  Bus Selector3/13 -> Scope2/1  "<psi_temp_const>"
  Bus Selector3/3 -> To Workspace18/1  "<range_id_X>"
  Bus Selector3/4 -> To Workspace19/1  "<range_iq_X>"
  Bus Selector3/5 -> To Workspace20/1  "<range_psid_Y>"
  Bus Selector3/6 -> To Workspace21/1  "<range_psiq_Y>"
  Bus Selector3/7 -> To Workspace22/1  "<range_id_Y>"
  Bus Selector3/8 -> To Workspace23/1  "<range_iq_Y>"
  Bus Selector3/9 -> To Workspace24/1  "<psiq_grid>"
  Bus Selector3/10 -> To Workspace25/1  "<psid_grid>"
  Bus Selector3/11 -> To Workspace26/1  "<id_grid>"
  Bus Selector3/12 -> To Workspace27/1  "<iq_grid>"
  Subsystem Reference/7 -> [AutoRefCurrentsConfig]
  [AutoRefCurrentsConfig] -> Bus Selector7/1, AutoRefCurrents/3(AutoRefCurrentsConfig)
  AutoRefCurrents/1(AutoRefCurrents_state_output) -> Bus Selector4/1
  Bus Selector4/1 -> Switch3/1  "<d>"
  Bus Selector4/2 -> Switch2/1  "<q>"
  Bus Selector7/1 -> Switch2/2, Switch3/2  "<enableCRS>"
  [ControlFlags] -> AutoRefCurrents/4(ControlFlags)
  [enteredOnlineID] -> Delay9/1
  OnlineID_subsystem/2 -> [enteredOnlineID]
  [TwoMassID_output] -> FOC/9(TwoMassID_output)
  Bus Selector/4 -> To Workspace1/1  "<measArrayTorque>"
  Bus Selector/5 -> To Workspace2/1  "<measArraySpeed>"
  dqTrans/1(ActualValues_corr) -> [ActualValues], Bus Selector1/1
  [GlobalConfig] -> FOC/8(GlobalConfig)
  Bus Selector8/1 -> To Workspace3/1  "<psi_array>"
  Delay/1 -> Subsystem Reference1/2
  Delay7/1 -> Subsystem Reference1/3
  Delay3/1 -> Subsystem Reference1/4
  Delay4/1 -> Subsystem Reference1/5
  Delay1/1 -> Subsystem Reference1/6
  Delay5/1 -> Subsystem Reference1/7
  Delay6/1 -> Subsystem Reference1/8
  Delay2/1 -> Subsystem Reference1/9
  Delay9/1 -> Subsystem Reference1/10
  Delay14/1 -> Subsystem Reference1/11
  Delay8/1 -> Subsystem Reference1/12
  Subsystem Reference1/1 -> [GlobalConfig]
  Subsystem Reference1/2 -> [ControlFlags]
  [GlobalConfig_in] -> Subsystem Reference1/1

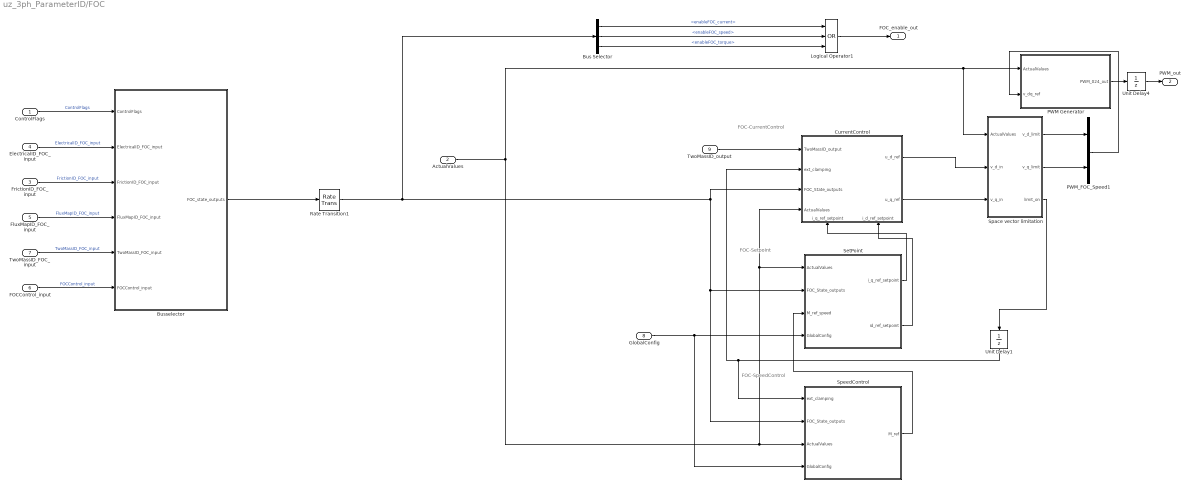
== system uz_3ph_ParameterID/FOC ==
  note: FOC-SpeedControl
  note: FOC-CurrentControl
  note: FOC-Setpoint
  ControlFlags : Inport
  ActualValues : Inport  Port=2
  FrictionID_FOC_input : Inport  Port=3
  ElectricalID_FOC_input : Inport  Port=4
  FluxMapID_FOC_input : Inport  Port=5
  FOCControl_input : Inport  Port=6
  TwoMassID_FOC_input : Inport  Port=7
  GlobalConfig : Inport  Port=8  OutDataTypeStr=Bus: uz_ParaID_GlobalConfig_t
  TwoMassID_output : Inport  Port=9  OutDataTypeStr=Bus: uz_ParaID_TwoMassID_output_t
  Bus Selector : BusSelector  OutputSignals=enableFOC_current,enableFOC_speed,enableFOC_torque
  Busselector : MATLAB Function  TreatAsAtomicUnit=on
  CurrentControl : Subsystem
      settings: PortSchema="{\"entries\":[{\"content\":{\"sides\":[{\"content\":{\"connectorIds\":[\"In1\",\"In2\",\"In3\",\"In4\"]},\"type\":\"ConnectorPlacement.EquallySpacedRectSide\",\"uuid\":\"77c09fd7-fff9-4bf9-9e3c-ae7d8d4ae844\"},{\"content\":{\"connectorIds\":[\"Out1\",\"Out2\"],\"side\":\"RIGHT\"},\"type\":\"ConnectorPlacement.EquallySpacedRectSide\",\"uuid\":\"d9a85257-d7d2-47a7-af12-4b0d4d0582bd\"},{\"content\":{\"connectorIds\":[],\"side\":\"TOP\"},\"type\":\"ConnectorPlacement.EquallySpacedRectSide\",\"uuid\":\"c30896ce-cf5a-4a2d-9d70-70e47f59ac53\"},{\"content\":{\"connectorIds\":[\"In5\",\"In6\"],\"side\":\"BOTTOM\"},\"type\":\"ConnectorPlacement.EquallySpacedRectSide\",\"uuid\":\"4956357e-f10e-445a-971a-b0f87868dbb6\"}]},\"type\":\"ConnectorPlacement.EquallySpacedConnector\",\"uuid\":\"e52ebb7a-573d-4053-a7f6-74acae9243d3\"}],\"packageUris\":[\"http://schema.mathworks.com/mf0/Connector/R2020b\"],\"version\":\"1.0\"}"
  Logical Operator1 : Logic  Operator=OR  Inputs=3  AllPortsSameDT=off  OutDataTypeStr=boolean
  PWM Generator : Subsystem
  PWM_FOC_Speed1 : Mux  Inputs=2
  Rate Transition1 : RateTransition  OutPortSampleTime=1/d_f_hardware
  SetPoint : Subsystem
  Space vector limitation : MATLAB Function  TreatAsAtomicUnit=on
  SpeedControl : Subsystem
  Unit Delay1 : UnitDelay  SampleTime=-1  HasFrameUpgradeWarning=on
  Unit Delay4 : UnitDelay  SampleTime=-1  HasFrameUpgradeWarning=on
  FOC_enable_out : Outport
  PWM_out : Outport  Port=2
  wires:
  FrictionID_FOC_input/1 -> Busselector/3(FrictionID_FOC_input)  "FrictionID_FOC_input"
  Bus Selector/1 -> Logical Operator1/1  "<enableFOC_current>"
  Bus Selector/2 -> Logical Operator1/2  "<enableFOC_speed>"
  FOCControl_input/1 -> Busselector/6(FOCControl_input)  "FOCControl_input"
  TwoMassID_FOC_input/1 -> Busselector/5(TwoMassID_FOC_input)  "TwoMassID_FOC_input"
  FluxMapID_FOC_input/1 -> Busselector/4(FluxMapID_FOC_input)  "FluxMapID_FOC_input"
  Rate Transition1/1 -> Bus Selector/1, SpeedControl/2(FOC_State_outputs), SetPoint/2(FOC_State_outputs), CurrentControl/3(FOC_State_outputs)
  ElectricalID_FOC_input/1 -> Busselector/2(ElectricalID_FOC_input)  "ElectricalID_FOC_input"
  ControlFlags/1 -> Busselector/1(ControlFlags)  "ControlFlags"
  PWM Generator/1(PWM_024_out) -> Unit Delay4/1
  Unit Delay4/1 -> PWM_out/1
  Logical Operator1/1 -> FOC_enable_out/1
  CurrentControl/1(u_d_ref) -> Space vector limitation/2(v_d_in)
  CurrentControl/2(u_q_ref) -> Space vector limitation/3(v_q_in)
  Space vector limitation/2(v_q_limit) -> PWM_FOC_Speed1/2
  Space vector limitation/1(v_d_limit) -> PWM_FOC_Speed1/1
  Space vector limitation/3(limit_on) -> Unit Delay1/1
  Unit Delay1/1 -> SpeedControl/1(ext_clamping), CurrentControl/2(ext_clamping)
  PWM_FOC_Speed1/1 -> PWM Generator/2(v_dq_ref)
  Busselector/1(FOC_state_outputs) -> Rate Transition1/1
  SetPoint/2(id_ref_setpoint) -> CurrentControl/6(i_d_ref_setpoint)
  SpeedControl/1(M_ref) -> SetPoint/3(M_ref_speed)
  ActualValues/1 -> Space vector limitation/1(ActualValues), PWM Generator/1(ActualValues), CurrentControl/4(ActualValues), SetPoint/1(ActualValues), SpeedControl/3(ActualValues)
  SetPoint/1(i_q_ref_setpoint) -> CurrentControl/5(i_q_ref_setpoint)
  GlobalConfig/1 -> SetPoint/4(GlobalConfig), SpeedControl/4(GlobalConfig)
  Bus Selector/3 -> Logical Operator1/3  "<enableFOC_torque>"
  TwoMassID_output/1 -> CurrentControl/1(TwoMassID_output)
